simulink model "InvertedPendulumLIN"  (R2017a)
settings: Solver=VariableStepAuto  StartTime=0.0  StopTime=10000  RelTol=1e-3
libraries: simulink x1
settings Model: Creator=aposad31  LastModifiedBy=santiago
settings OptimizationCC: BlockReduction=off  DefaultParameterBehavior=Inlined  BufferReuse=off

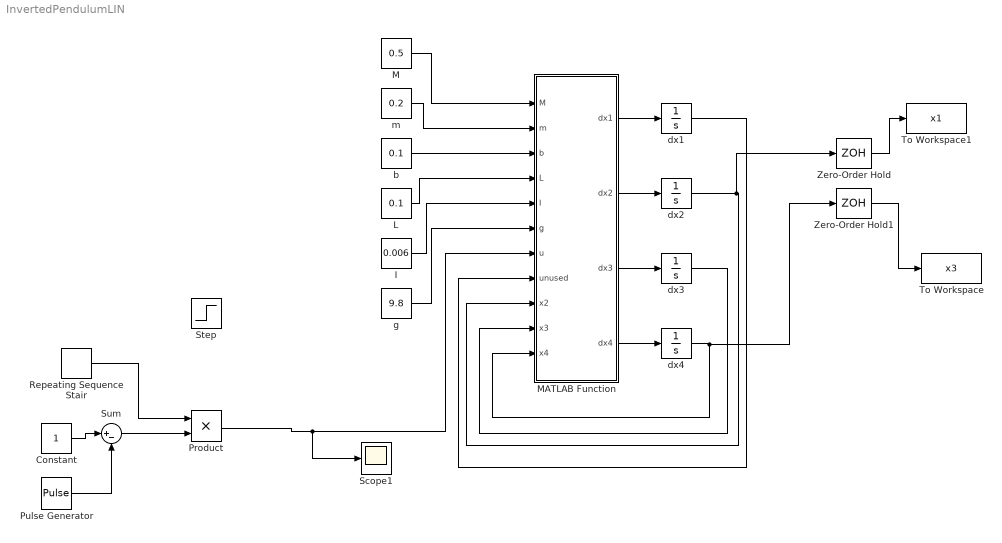
== system InvertedPendulumLIN ==
  Constant : Constant
  I : Constant  Value=0.006
  L : Constant  Value=0.1
  M : Constant  Value=0.5
  MATLAB Function : MATLAB Function  TreatAsAtomicUnit=on
  Product : Product
  Pulse Generator : DiscretePulseGenerator  PulseType=Time based  Period=100  PulseWidth=90
  Repeating Sequence Stair : simulink/Sources/Repeating Sequence Stair  OutValues=-5:0.1:5  tsamp=100  OutMin=[]  OutMax=[]  OutDataTypeStr=double  OutputDataTypeScalingMode=double  OutDataType=fixdt(0,8)  ConRadixGroup=Best Precision: Vector-wise  OutScaling=2^-12
  Scope1 : Scope
  Step : Step  After=-5  SampleTime=0
  Sum : Sum  Inputs=|+-
  To Workspace : ToWorkspace  VariableName=x3  SaveFormat=Timeseries  SampleTime=-1
  To Workspace1 : ToWorkspace  VariableName=x1  SaveFormat=Timeseries  SampleTime=-1
  Zero-Order Hold : ZeroOrderHold  SampleTime=300
  Zero-Order Hold1 : ZeroOrderHold  SampleTime=100
  b : Constant  Value=0.1
  dx{1..4} (4 alike) : Integrator
  g : Constant  Value=9.8
  m : Constant  Value=0.2
  wires:
  dx3/1 -> MATLAB Function/10(x3)
  dx1/1 -> MATLAB Function/8(unused)
  I/1 -> MATLAB Function/5(I)
  L/1 -> MATLAB Function/4(L)
  g/1 -> MATLAB Function/6(g)
  dx2/1 -> Zero-Order Hold/1, MATLAB Function/9(x2)
  MATLAB Function/4(dx4) -> dx4/1
  b/1 -> MATLAB Function/3(b)
  M/1 -> MATLAB Function/1(M)
  MATLAB Function/3(dx3) -> dx3/1
  dx4/1 -> Zero-Order Hold1/1, MATLAB Function/11(x4)
  MATLAB Function/1(dx1) -> dx1/1
  m/1 -> MATLAB Function/2(m)
  MATLAB Function/2(dx2) -> dx2/1
  Repeating Sequence Stair/1 -> Product/1
  Zero-Order Hold1/1 -> To Workspace/1
  Product/1 -> Scope1/1, MATLAB Function/7(u)
  Sum/1 -> Product/2
  Pulse Generator/1 -> Sum/2
  Constant/1 -> Sum/1
  Zero-Order Hold/1 -> To Workspace1/1

== matlab function InvertedPendulumLIN/MATLAB Function ==
  data: M input; m input; b input; L input; I input; g input; u input; dx1 output; unused input; x2 input; x3 input; x4 input; dx2 output; dx3 output; dx4 output
function [dx1, dx2, dx3, dx4] = fcn(M, m, b, L, I, g, u, ~, x2, x3, x4)
    denominator = (M+m).*(I+m.*L.^2)-m.^2.*L.^2.*cos(x3).^2;
    dx1 = x2;
    dx2 = ((I+m.*L.^2).*(u-b.*x2+m.*L.*x4.^2.*sin(x3))+m.^2.*L.^2.*g.*sin(x3).*cos(x3))./denominator;
    dx3 = x4;
    dx4 = (-m.*L.*u.*cos(x3)+m.*L.*b.*x2.*cos(x3)-m.^2.*L.^2.*x4.^2.*sin(x3).*cos(x3)-(M+m).*m*g.*L.*sin(x3))./denominator;
end
